simulink model "my_pv_system_1_sm_master"  (Simulink 8.4)
settings: Solver=ode3  StartTime=0.0  StopTime=inf  FixedStep=5e-05  RelTol=1e-3
undefined symbols (not defined in the file or in its folder): another_event_name, my_event_name
libraries: powerlib x31, opal_lib x8, powerlib_meascontrol x2, rtlab x1
Description:
  | Model of a simple control system for use iin training.
settings Model: Creator=Paul Baracos  LastModifiedBy=jiang  BufferReuse=off
settings DataIOCC: SaveOutput=off  SaveTime=off  SignalLoggingName=sigsOut
settings OptimizationCC: BlockReduction=off  BooleanDataType=off  OptimizeBlockIOStorage=off  BufferReuse=off  GlobalBufferReuse=off  ExpressionFolding=off  ExpressionDepthLimit=128  LocalBlockOutputs=off  InitFltsAndDblsToZero=on
settings DebuggingCC: SaveWithParameterizedLinksMsg=none  SignalResolutionControl=TryResolveAllWithWarning  SolverPrmCheckMsg=none  MultiTaskDSMMsg=warning  MultiTaskCondExecSysMsg=none  StateNameClashWarn=none
settings HardwareCC: TargetHWDeviceType=32-bit Generic  TargetUnknown=on  ProdEqTarget=off
settings RTWCC: GenCodeOnly=on  IncludeERTFirstTime=on
settings GRTTargetCC: TargetFcnLib=ansi_tfl_tmw.mat

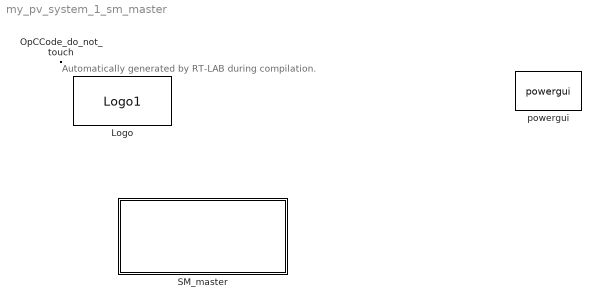
== system my_pv_system_1_sm_master ==
  note: Automatically generated by RT-LAB during compilation.
  Logo : opal_lib/Logo1  vide=[]
  OpCCode_do_not_touch : opal_lib/Communication/OpCCode  SystemSampleTime=-1
  SM_master : Subsystem
  powergui : powerlib/powergui  SimulationMode=Discrete  SolverType=Tustin/Backward Euler (TBE)  SampleTime=5e-05  frequency=60  SPID=off  DisableSnubberDevices=off  DisableRonSwitches=off  DisableVfSwitches=off  SwTol=0  DisplayEquations=off  Interpol=off  methode=off  Ts=100  frequencyindice=50  Pbase=100e6  ErrMax=1e-4  Iterations=50  UnitsV=kV  UnitsW=MW  FunctionMessages=off  echomessages=off  HookPort=off  EnableUseOfTLC=off  x0status=blocks  RestoreLinks=warning  ResistiveCurrentMeasurement=off  Frange=[0:2:500]  Ylog=off  Xlog=on  ShowGrid=off  save=off  variable=ZData  structure=0  ZoomFFT=off  StartTime=0.0  cycles=1  DisplayStyle=1  fundamental=60  FreqAxis=off  MaxFrequency=1000  frequencyindicesteady=1  RmsSteady=1  display=off

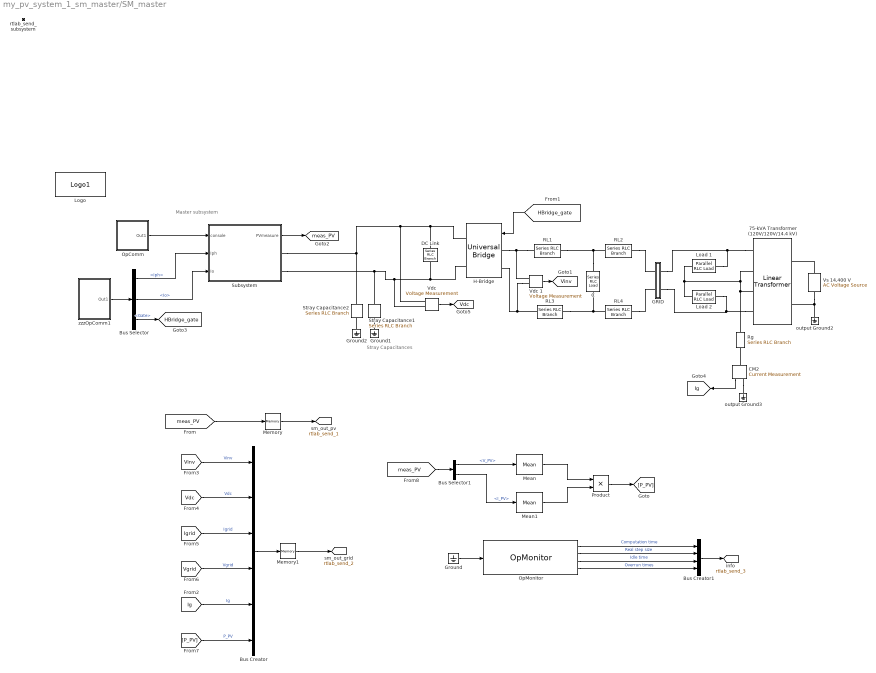
== system my_pv_system_1_sm_master/SM_master ==
  note: Master subsystem
  note: Stray
      | Capacitances
  75-kVA Transformer (120V/120V/14.4 kV) : powerlib/Elements/Linear Transformer  UNITS=pu  NominalPower=[75e3,60]  winding1=[14.4e3 0.01,0.03]  winding2=[120,0.02,0]  ThreeWindings=on  winding3=[120,0.02,0]  RmLm=[50,50]  Measurements=None  DataType=off
  Bus Creator : BusCreator  Inputs=6
  Bus Creator1 : BusCreator
  Bus Selector : BusSelector  OutputSignals=Iph,Io,Gate
  Bus Selector1 : BusSelector  OutputSignals=V_PV,I_PV
  C : powerlib/Elements/Series RLC Load  LConnTagsString=a  RConnTagsString=__new0  NominalVoltage=240  NominalFrequency=60  ActivePower=10.5  InductivePower=0  CapacitivePower=525  Setx0=off  InitialVoltage=0  SetiL0=off  InitialCurrent=0  Measurements=None
  CM2 : powerlib/Measurements/Current Measurement  PhasorSimulation=off  OutputType=Complex  PSBequivalent=0
  DC Link : powerlib/Elements/Series RLC Branch  LConnTagsString=__new0  RConnTagsString=__new0  BranchType=C  Resistance=1.0  Inductance=1.0  SetiL0=off  InitialCurrent=0  Capacitance=3000e-6  Setx0=on  InitialVoltage=425  Measurements=None
  GRID : Subsystem
  Ground : Ground
  Ground1 : powerlib/Elements/Ground  LConnTagsString=a
  Ground2 : powerlib/Elements/Ground  LConnTagsString=a
  "H-Bridge " : powerlib/Power Electronics/Universal Bridge  Arms=2  SnubberResistance=1e6  SnubberCapacitance=inf  Device=IGBT / Diodes  Ron=1e-3  Lon=0  ForwardVoltages=[ 0 0 ]  ForwardVoltage=0  GTOparameters=[ 10e-6 , 20e-6 ]  IGBTparameters=[ 50e-6 , 50e-6 ]*0  Measurements=None  Measurements_2=None  converterType=Rectifier
  Load 1 : powerlib/Elements/Parallel RLC Load  LConnTagsString=a  RConnTagsString=__new0  NominalVoltage=120  NominalFrequency=50  ActivePower=5e3  InductivePower=2e3  CapacitivePower=0  Setx0=off  InitialVoltage=0  SetiL0=off  InitialCurrent=0  Measurements=None
      settings: AttributesFormatString=\n
  Load 2 : powerlib/Elements/Parallel RLC Load  LConnTagsString=a  RConnTagsString=__new0  NominalVoltage=120  NominalFrequency=50  ActivePower=5e3  InductivePower=2e3  CapacitivePower=0  Setx0=off  InitialVoltage=0  SetiL0=off  InitialCurrent=0  Measurements=None
      settings: AttributesFormatString=\n
  Logo : opal_lib/Logo1  vide=[]
  Mean : powerlib_meascontrol/Measurements/Mean  Freq=50  Vinit=0  Ts=0
  Mean1 : powerlib_meascontrol/Measurements/Mean  Freq=50  Vinit=0  Ts=0
  Memory : Memory  InheritSampleTime=on
  Memory1 : Memory  InheritSampleTime=on
  OpComm : Subsystem
      mask init:
      | opmaskdisplay('maskdisplay_block',gcb,'disp(''OpComm'')');
      mask Display:
      | patch([0 0.5 0.7 0],[1 1 0 0],[0.7 0.75 0.9]);
      | patch([1 0.53 0.73 1],[1 1 0 0],[1 0.8 0.7]);
      | plot([0 0 1 1 0],[0 1 1 0 0]);
      | disp('OpComm')
  OpMonitor : rtlab/Monitoring/OpMonitor  compute_time=on  real_step=on  idle_time=on  nb_overruns=on  user_time=off  user_name=my_event_name,another_event_name
  Product : Product
  RL{1..4} (4 alike) : powerlib/Elements/Series RLC Branch  LConnTagsString=__new0  RConnTagsString=__new0  BranchType=RL  Resistance=8.23e-3  Inductance=2.183e-3  SetiL0=off  InitialCurrent=0  Capacitance=1e-6  Setx0=off  InitialVoltage=0  Measurements=None
  Rg : powerlib/Elements/Series RLC Branch  LConnTagsString=__new0  RConnTagsString=__new0  BranchType=R  Resistance=0.2  Inductance=1  SetiL0=off  InitialCurrent=0  Capacitance=50e-9  Setx0=off  InitialVoltage=0  Measurements=None
  Stray Capacitance1 : powerlib/Elements/Series RLC Branch  LConnTagsString=__new0  RConnTagsString=__new0  BranchType=C  Resistance=1e-3  Inductance=1  SetiL0=off  InitialCurrent=0  Capacitance=4e-9  Setx0=off  InitialVoltage=0  Measurements=None
  Stray Capacitance2 : powerlib/Elements/Series RLC Branch  LConnTagsString=__new0  RConnTagsString=__new0  BranchType=C  Resistance=1e-3  Inductance=1  SetiL0=off  InitialCurrent=0  Capacitance=4e-9  Setx0=off  InitialVoltage=0  Measurements=None
  Subsystem : Subsystem
  "Vdc " : powerlib/Measurements/Voltage Measurement  Tag=PoWeRsYsTeMmEaSuReMeNt  PhasorSimulation=off  OutputType=Magnitude  PSBequivalent=0
  Vdc 1 : powerlib/Measurements/Voltage Measurement  Tag=PoWeRsYsTeMmEaSuReMeNt  PhasorSimulation=off  OutputType=Magnitude  PSBequivalent=0
  Vs 14,400 V : powerlib/Electrical Sources/AC Voltage Source  Description=source block  Amplitude=14400*sqrt(2)  Phase=0  Frequency=50  SampleTime=0  Measurements=None
      settings: AttributesFormatString=\n
  output Ground2 : powerlib/Elements/Ground  LConnTagsString=a
  output Ground3 : powerlib/Elements/Ground  LConnTagsString=a
  rtlab_send_subsystem : Subsystem  Priority=-100
      mask Display: text(0,0,'');
  zzzOpComm1 : Subsystem
      mask init:
      | opmaskdisplay('maskdisplay_block',gcb,'disp(''OpComm'')');
      mask Display:
      | patch([0 0.5 0.7 0],[1 1 0 0],[0.7 0.75 0.9]);
      | patch([1 0.53 0.73 1],[1 1 0 0],[1 0.8 0.7]);
      | plot([0 0 1 1 0],[0 1 1 0 0]);
      | disp('OpComm')
  tag scope: HBridge_gate=global, Ig=global, Vdc=global, Vinv=global, meas_PV=global, rtlab_send_1=global, rtlab_send_2=global, rtlab_send_3=global
  wires:
  Memory/1 -> [rtlab_send_1]
  Vdc 1/1 -> [Vinv]
  "Vdc "/1 -> [Vdc]
  Subsystem/1(PVmeasure) -> [meas_PV]
  [meas_PV] -> Memory/1
  [HBridge_gate] -> "H-Bridge "/1
  CM2/1 -> [Ig]
  Memory1/1 -> [rtlab_send_2]
  [Vinv] -> Bus Creator/1  "Vinv"
  [Vdc] -> Bus Creator/2  "Vdc"
  [Igrid] -> Bus Creator/3  "Igrid"
  [Vgrid] -> Bus Creator/4  "Vgrid"
  [Ig] -> Bus Creator/5  "Ig"
  Bus Creator/1 -> Memory1/1
  OpComm/1(Out1) -> Subsystem/1(console)
  zzzOpComm1/1(Out1) -> Bus Selector/1
  Bus Selector/1 -> Subsystem/2(Iph)  "<Iph>"
  Bus Selector/2 -> Subsystem/3(Io)  "<Io>"
  Bus Selector/3 -> [HBridge_gate]  "<Gate>"
  Bus Creator1/1 -> [rtlab_send_3]
  OpMonitor/3 -> Bus Creator1/3  "Idle time"
  OpMonitor/1 -> Bus Creator1/1  "Computation time"
  OpMonitor/2 -> Bus Creator1/2  "Real step size"
  OpMonitor/4 -> Bus Creator1/4  "Overrun times"
  Ground/1 -> OpMonitor/1
  [meas_PV] -> Bus Selector1/1
  Bus Selector1/1 -> Mean/1  "<V_PV>"
  Bus Selector1/2 -> Mean1/1  "<I_PV>"
  Mean/1 -> Product/1
  Mean1/1 -> Product/2
  Product/1 -> [P_PV]
  [P_PV] -> Bus Creator/6  "P_PV"
  connections:
  Subsystem/RConn1 -- Stray Capacitance2/LConn1 -- "Vdc "/LConn1 -- DC Link/LConn1 -- "H-Bridge "/RConn1
  RL1/LConn1 -- "H-Bridge "/LConn1 -- Vdc 1/LConn1
  Vdc 1/LConn2 -- "H-Bridge "/LConn2 -- RL3/LConn1
  C/RConn1 -- RL1/RConn1 -- RL2/LConn1
  RL4/LConn1 -- C/LConn1 -- RL3/RConn1
  DC Link/RConn1 -- "H-Bridge "/RConn2 -- Stray Capacitance1/LConn1 -- Subsystem/RConn2 -- "Vdc "/LConn2
  75-kVA Transformer (120V/120V/14.4 kV)/LConn2 -- output Ground2/LConn1 -- Vs 14,400 V/LConn1
  75-kVA Transformer (120V/120V/14.4 kV)/RConn4 -- Load 2/RConn1 -- GRID/RConn2
  75-kVA Transformer (120V/120V/14.4 kV)/RConn1 -- Load 1/RConn1 -- GRID/RConn1
  Load 2/LConn1 -- Load 1/LConn1 -- 75-kVA Transformer (120V/120V/14.4 kV)/RConn2 -- Rg/LConn1 -- 75-kVA Transformer (120V/120V/14.4 kV)/RConn3
  RL2/RConn1 -- GRID/LConn1
  RL4/RConn1 -- GRID/LConn2
  Ground2/LConn1 -- Stray Capacitance2/RConn1
  Vs 14,400 V/RConn1 -- 75-kVA Transformer (120V/120V/14.4 kV)/LConn1
  Ground1/LConn1 -- Stray Capacitance1/RConn1
  CM2/RConn1 -- output Ground3/LConn1
  CM2/LConn1 -- Rg/RConn1

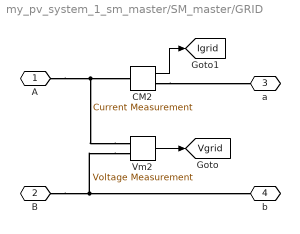
== system my_pv_system_1_sm_master/SM_master/GRID ==
  CM2 : powerlib/Measurements/Current Measurement  PhasorSimulation=off  OutputType=Complex  PSBequivalent=0
  Vm2 : powerlib/Measurements/Voltage Measurement  PhasorSimulation=off  OutputType=Complex  PSBequivalent=0
  A : PMIOPort  Port=1  Side=Left
  B : PMIOPort  Port=2  Side=Left
  a : PMIOPort  Port=3  Side=Right
  b : PMIOPort  Port=4  Side=Right
  tag scope: Igrid=global, Vgrid=global
  wires:
  Vm2/1 -> [Vgrid]
  CM2/1 -> [Igrid]
  connections:
  Vm2/LConn2 -- b/RConn1 -- B/RConn1
  Vm2/LConn1 -- A/RConn1 -- CM2/LConn1
  CM2/RConn1 -- a/RConn1

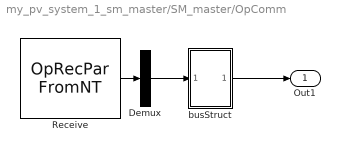
== system my_pv_system_1_sm_master/SM_master/OpComm ==
  Demux : Demux  Outputs=[2]
  Receive : opal_lib/Communication/OpRecPar FromNT  Data_width=2  InitialConditions=[1000;25]
  busStruct : Subsystem
  Out1 : Outport
  wires:
  Demux/1 -> busStruct/1(In1)
  busStruct/1(Out1) -> Out1/1
  Receive/1 -> Demux/1

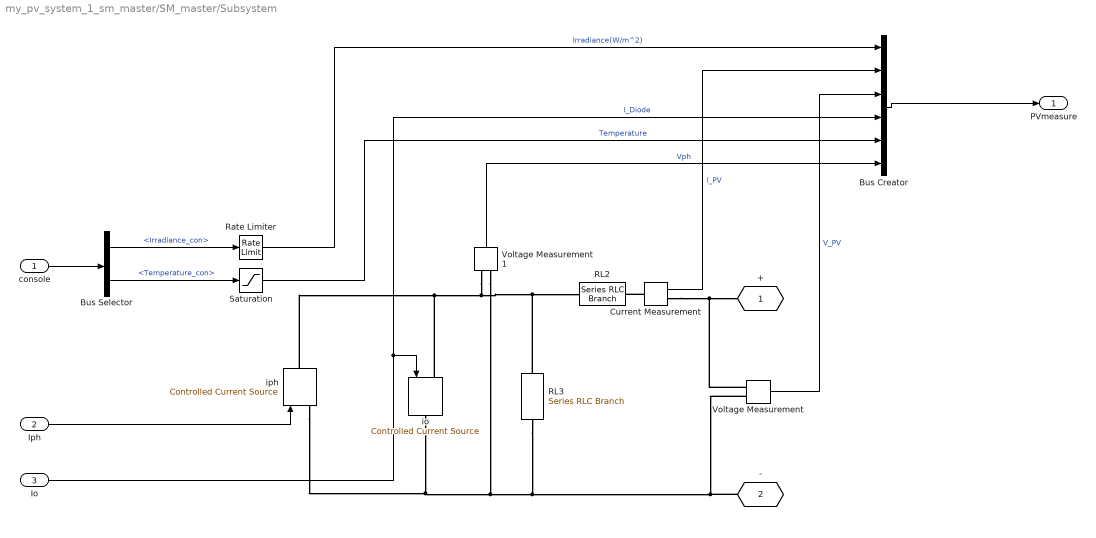
== system my_pv_system_1_sm_master/SM_master/Subsystem ==
  console : Inport
  Iph : Inport  Port=2
  Io : Inport  Port=3
  Bus Creator : BusCreator  Inputs=6
  Bus Selector : BusSelector  OutputSignals=Irradiance_con,Temperature_con
  Current Measurement : powerlib/Measurements/Current Measurement  PhasorSimulation=off  OutputType=Complex  PSBequivalent=0
  RL2 : powerlib/Elements/Series RLC Branch  LConnTagsString=__new0  RConnTagsString=__new0  BranchType=R  Resistance=0.247*14  Inductance=2.183e-3  SetiL0=off  InitialCurrent=0  Capacitance=1e-6  Setx0=off  InitialVoltage=0  Measurements=None
  RL3 : powerlib/Elements/Series RLC Branch  LConnTagsString=__new0  RConnTagsString=__new0  BranchType=R  Resistance=301.8*14  Inductance=2.183e-3  SetiL0=off  InitialCurrent=0  Capacitance=1e-6  Setx0=off  InitialVoltage=0  Measurements=None
  Rate Limiter : RateLimiter  RisingSlewLimit=8000  FallingSlewLimit=-8000  SampleTimeMode=inherited  InitialCondition=1000
  Saturation : Saturate  UpperLimit=55  LowerLimit=5
  Voltage Measurement : powerlib/Measurements/Voltage Measurement  PhasorSimulation=off  OutputType=Complex  PSBequivalent=0
  Voltage Measurement1 : powerlib/Measurements/Voltage Measurement  PhasorSimulation=off  OutputType=Complex  PSBequivalent=0
  "io " : powerlib/Electrical Sources/Controlled Current Source  Initialize=on  Source_Type=DC  Amplitude=8.05  Phase=0  Frequency=0  Measurements=None
  "iph " : powerlib/Electrical Sources/Controlled Current Source  Initialize=on  Source_Type=DC  Amplitude=8.05  Phase=0  Frequency=0  Measurements=None
  + : PMIOPort  Port=1  Side=Right
  - : PMIOPort  Port=2  Side=Right
  PVmeasure : Outport
  wires:
  Voltage Measurement/1 -> Bus Creator/3  "V_PV"
  Current Measurement/1 -> Bus Creator/2  "I_PV"
  Bus Creator/1 -> PVmeasure/1
  Io/1 -> Bus Creator/4, "io "/1  "I_Diode"
  console/1 -> Bus Selector/1
  Iph/1 -> "iph "/1
  Voltage Measurement1/1 -> Bus Creator/6  "Vph"
  Bus Selector/1 -> Rate Limiter/1  "<Irradiance_con>"
  Bus Selector/2 -> Saturation/1  "<Temperature_con>"
  Rate Limiter/1 -> Bus Creator/1  "Irradiance(W/m^2)"
  Saturation/1 -> Bus Creator/5  "Temperature"
  connections:
  "iph "/RConn1 -- "io "/LConn1 -- RL3/RConn1 -- RL2/LConn1 -- Voltage Measurement1/LConn1
  "io "/RConn1 -- "iph "/LConn1 -- Voltage Measurement/LConn2 -- -/RConn1 -- RL3/LConn1 -- Voltage Measurement1/LConn2
  Current Measurement/LConn1 -- RL2/RConn1
  Current Measurement/RConn1 -- Voltage Measurement/LConn1 -- +/RConn1

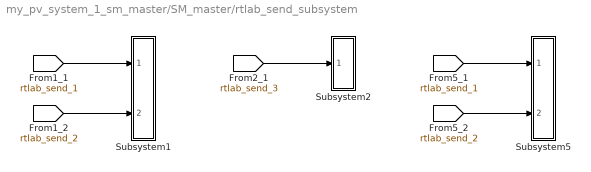
== system my_pv_system_1_sm_master/SM_master/rtlab_send_subsystem ==
  Subsystem1 : Subsystem
  Subsystem2 : Subsystem
  Subsystem5 : Subsystem  Priority=-200000  TreatAsAtomicUnit=on
  wires:
  [rtlab_send_1] -> Subsystem1/1(In1)
  [rtlab_send_2] -> Subsystem1/2(In2)
  [rtlab_send_3] -> Subsystem2/1(In1)
  [rtlab_send_1] -> Subsystem5/1(In1)
  [rtlab_send_2] -> Subsystem5/2(In2)

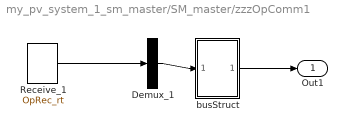
== system my_pv_system_1_sm_master/SM_master/zzzOpComm1 ==
  Demux_1 : Demux  Outputs=[6]
  Receive_1 : opal_lib/Communication/OpRec_rt  src=3  Data_width=6  st=5e-05
  busStruct : Subsystem
  Out1 : Outport
  wires:
  Demux_1/1 -> busStruct/1(In1)
  busStruct/1(Out1) -> Out1/1
  Receive_1/1 -> Demux_1/1

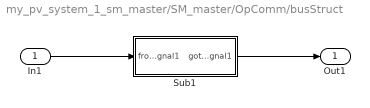
== system my_pv_system_1_sm_master/SM_master/OpComm/busStruct ==
  In1 : Inport
  Sub1 : Subsystem
  Out1 : Outport
  wires:
  Sub1/1(goto_signal1) -> Out1/1
  In1/1 -> Sub1/1(from_signal1)

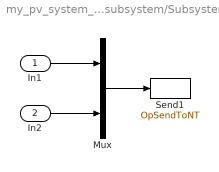
== system my_pv_system_1_sm_master/SM_master/rtlab_send_subsystem/Subsystem1 ==
  In1 : Inport
  In2 : Inport  Port=2
  Mux : Mux  Inputs=2
  Send1 : opal_lib/Communication/OpSendToNT  Acqu_group=1
  wires:
  Mux/1 -> Send1/1
  In1/1 -> Mux/1
  In2/1 -> Mux/2

== system my_pv_system_1_sm_master/SM_master/rtlab_send_subsystem/Subsystem2 ==
  In1 : Inport
  Mux : Mux  Inputs=1
  Send2 : opal_lib/Communication/OpSendToNT  Acqu_group=2
  wires:
  Mux/1 -> Send2/1
  In1/1 -> Mux/1

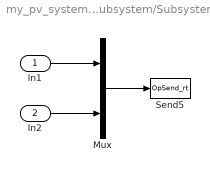
== system my_pv_system_1_sm_master/SM_master/rtlab_send_subsystem/Subsystem5 ==
  In1 : Inport
  In2 : Inport  Port=2
  Mux : Mux  Inputs=2
  Send5 : opal_lib/Communication/OpSend_rt  dest=3  priority2=0  st=5e-05
  wires:
  Mux/1 -> Send5/1
  In1/1 -> Mux/1
  In2/1 -> Mux/2

== system my_pv_system_1_sm_master/SM_master/zzzOpComm1/busStruct ==
  In1 : Inport
  Sub1 : Subsystem
  Out1 : Outport
  wires:
  Sub1/1(goto_signal1) -> Out1/1
  In1/1 -> Sub1/1(from_signal1)

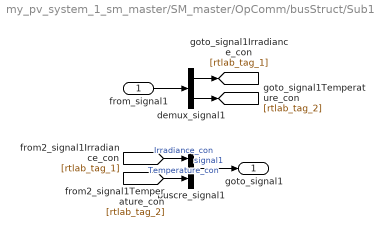
== system my_pv_system_1_sm_master/SM_master/OpComm/busStruct/Sub1 ==
  from_signal1 : Inport
  buscre_signal1 : BusCreator  Inputs=2
  demux_signal1 : Demux  Outputs="[1  1]"
  goto_signal1 : Outport
  wires:
  buscre_signal1/1 -> goto_signal1/1  "signal1"
  [rtlab_tag_2] -> buscre_signal1/2  "Temperature_con"
  [rtlab_tag_1] -> buscre_signal1/1  "Irradiance_con"
  demux_signal1/2 -> [rtlab_tag_2]
  demux_signal1/1 -> [rtlab_tag_1]
  from_signal1/1 -> demux_signal1/1

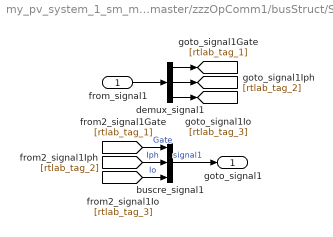
== system my_pv_system_1_sm_master/SM_master/zzzOpComm1/busStruct/Sub1 ==
  from_signal1 : Inport
  buscre_signal1 : BusCreator  Inputs=3
  demux_signal1 : Demux  Outputs="[4  1  1]"
  goto_signal1 : Outport
  wires:
  buscre_signal1/1 -> goto_signal1/1  "signal1"
  [rtlab_tag_3] -> buscre_signal1/3  "Io"
  [rtlab_tag_2] -> buscre_signal1/2  "Iph"
  [rtlab_tag_1] -> buscre_signal1/1  "Gate"
  demux_signal1/3 -> [rtlab_tag_3]
  demux_signal1/2 -> [rtlab_tag_2]
  demux_signal1/1 -> [rtlab_tag_1]
  from_signal1/1 -> demux_signal1/1
